simulink model "ModelNoStep1"  (R2013b)
settings: Solver=ode45  StartTime=0.0  StopTime=10.0  RelTol=1e-3
values from neighbouring files (symbols this model uses):
  D = xopt(3)    [Plant1delay.m]    (also in Plant2.m; Plant2delay.m; Plant3.m; Plant4.m)
  denum = [T1(i) 1]    [Plant1delay.m]    (also in Plant2.m = [1 1 1]; Plant2delay.m = [T2(i)*T2(i) 2*T2(i) 1]; Plant3.m = [T3(i)*T3(i) T3(i)*T3(i)+2*T3 2*T3(i) 1 1]; Plant8.m = [1 3 3 1])
  I = xopt(2)    [Plant1delay.m]    (also in Plant2.m; Plant2delay.m; Plant3.m; Plant4.m)
  N = xopt(4)    [Plant1delay.m]    (also in Plant2.m; Plant2delay.m; Plant3.m; Plant4.m)
  num = [1]    [Plant1delay.m]    (also in Plant2.m; Plant2delay.m; Plant3.m; Plant8.m = [-alfa8(i) 1])
  P = xopt(1)    [Plant1delay.m]    (also in Plant2.m; Plant2delay.m; Plant3.m; Plant4.m)
settings Model: Creator=stelmo  LastModifiedBy=stelmo

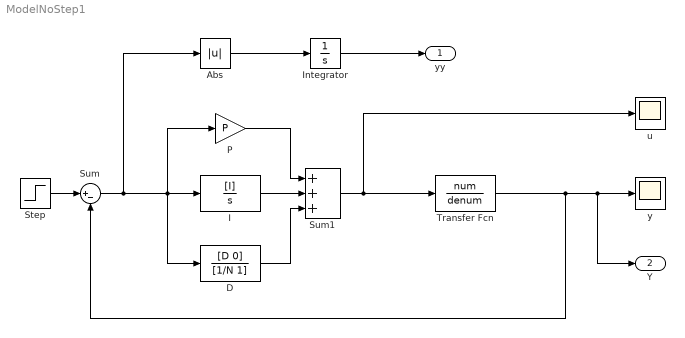
== system ModelNoStep1 ==
  Abs : Abs
  D : TransferFcn  Numerator=[D 0]  Denominator=[1/N 1]
  I : TransferFcn  Numerator=[I]  Denominator=[1 0]
  Integrator : Integrator
  P : Gain  Gain=P
  Step : Step  SampleTime=0
  Sum : Sum  Inputs=|+-
  Sum1 : Sum  Inputs=+++
  Transfer Fcn : TransferFcn  Numerator=num  Denominator=denum
  u : Scope
  y : Scope
      settings: MaxDataPoints=50000000
  yy : Outport
  Y : Outport  Port=2
  wires:
  Step/1 -> Sum/1
  Sum/1 -> D/1, P/1, I/1, Abs/1
  Transfer Fcn/1 -> Y/1, y/1, Sum/2
  Abs/1 -> Integrator/1
  Integrator/1 -> yy/1
  P/1 -> Sum1/1
  I/1 -> Sum1/2
  D/1 -> Sum1/3
  Sum1/1 -> Transfer Fcn/1, u/1
